simulink model "LinearVehicleiLQR"  (R2021a)
settings: Solver=FixedStepDiscrete  StartTime=0.0  StopTime=100  FixedStep=0.001  MaxStep=0.01  RelTol=1e-3
values from neighbouring files (symbols this model uses):
  Q = [1 0 0; 0 1 0; 0 0 10]    [LQR.m]    (also in NonlinearVehicleLQR.m = eye(3)*10; NonlinearVehicleiLQR.m = eye(3)*10; SringiLQR.m = [1 0; 0 1]*1; SringiLQR2.m = [1 0; 0 1]*1)
  Qf = eye(3)    [LQR.m]    (also in NonlinearVehicleLQR.m; NonlinearVehicleiLQR.m; SringiLQR.m = [1 0; 0 1]; SringiLQR2.m = [1 0; 0 1])
  R = eye(2)*10^-4    [LQR.m]    (also in NonlinearVehicleLQR.m = eye(2)*10^-2; NonlinearVehicleiLQR.m = eye(2)*10^-2; SringiLQR.m = eye(1)*1e-2; SringiLQR2.m = eye(1)*1e-2)
settings Model: Creator=iris  LastModifiedBy=iris
settings SolverCC: AlgebraicLoopSolver=TrustRegion
settings DebuggingCC: SFMachineParentedDataDiag=warning

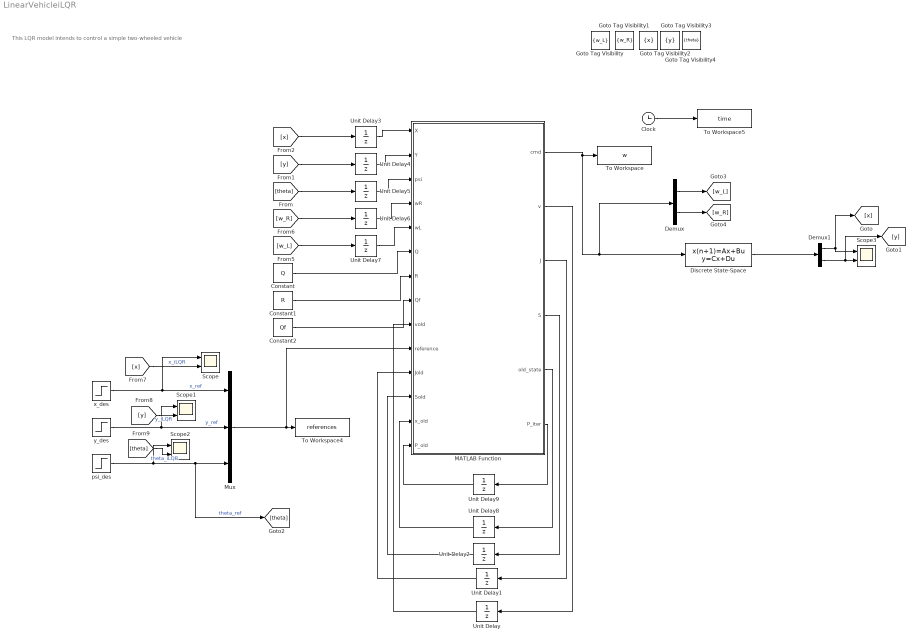
== system LinearVehicleiLQR ==
  note: This LQR model intends to control a simple two-wheeled vehicle
  Clock : Clock
  Constant : Constant  Value=Q
  Constant1 : Constant  Value=R
  Constant2 : Constant  Value=Qf
  Demux : Demux  Outputs=2
  Demux1 : Demux  Outputs=2
  Discrete State-Space : DiscreteStateSpace  A=eye(3)  B=[0.001 0;0 0; 0 0.001]  C=eye(3)  D=zeros(3,2)  SampleTime=-1
  Goto Tag Visibility : GotoTagVisibility  GotoTag=w_L
  Goto Tag Visibility1 : GotoTagVisibility  GotoTag=w_R
  Goto Tag Visibility2 : GotoTagVisibility  GotoTag=x
  Goto Tag Visibility3 : GotoTagVisibility  GotoTag=y
  Goto Tag Visibility4 : GotoTagVisibility  GotoTag=theta
  MATLAB Function : MATLAB Function  TreatAsAtomicUnit=on
  Mux : Mux  Inputs=3
  Scope{,1..3} (4 alike) : Scope  NumInputPorts=2
  To Workspace : ToWorkspace  VariableName=w  SampleTime=-1
  To Workspace4 : ToWorkspace  VariableName=references  SampleTime=-1
  To Workspace5 : ToWorkspace  VariableName=time  SampleTime=-1
  Unit Delay : UnitDelay  InitialCondition=zeros(2,1)  SampleTime=-1  HasFrameUpgradeWarning=on
  Unit Delay1 : UnitDelay  InitialCondition=10000  SampleTime=-1  HasFrameUpgradeWarning=on
  Unit Delay2 : UnitDelay  InitialCondition=Qf  SampleTime=-1  HasFrameUpgradeWarning=on
  Unit Delay{3..7} (5 alike) : UnitDelay  SampleTime=-1  HasFrameUpgradeWarning=on
  Unit Delay8 : UnitDelay  InitialCondition=[0,0]  SampleTime=-1  HasFrameUpgradeWarning=on
  Unit Delay9 : UnitDelay  InitialCondition=zeros(2)  SampleTime=-1  HasFrameUpgradeWarning=on
  psi_des : Step  Time=0  SampleTime=0
  x_des : Step  Time=0  SampleTime=0
  y_des : Step  Time=0  SampleTime=0
  wires:
  MATLAB Function/3(J) -> Unit Delay1/1
  Unit Delay1/1 -> MATLAB Function/11(Jold)
  MATLAB Function/4(S) -> Unit Delay2/1
  Unit Delay2/1 -> MATLAB Function/12(Sold)
  MATLAB Function/2(v) -> Unit Delay/1
  Unit Delay/1 -> MATLAB Function/9(vold)
  MATLAB Function/1(cmd) -> To Workspace/1, Demux/1, Discrete State-Space/1
  [theta] -> Unit Delay5/1
  [x] -> Unit Delay3/1
  [y] -> Unit Delay4/1
  [w_L] -> Unit Delay7/1
  [w_R] -> Unit Delay6/1
  Constant/1 -> MATLAB Function/6(Q)
  Constant1/1 -> MATLAB Function/7(R)
  Constant2/1 -> MATLAB Function/8(Qf)
  Mux/1 -> MATLAB Function/10(reference), To Workspace4/1
  y_des/1 -> Scope1/1, Mux/2  "y_ref"
  x_des/1 -> Mux/1, Scope/1  "x_ref"
  psi_des/1 -> Scope2/1, [theta], Mux/3  "theta_ref"
  Unit Delay3/1 -> MATLAB Function/1(X)
  Unit Delay4/1 -> MATLAB Function/2(Y)
  Unit Delay5/1 -> MATLAB Function/3(psi)
  Unit Delay6/1 -> MATLAB Function/4(wR)
  Unit Delay7/1 -> MATLAB Function/5(wL)
  Clock/1 -> To Workspace5/1
  [x] -> Scope/2  "x_iLQR"
  [y] -> Scope1/2  "y_iLQR"
  [theta] -> Scope2/2  "theta_iLQR"
  Discrete State-Space/1 -> Demux1/1
  Demux1/1 -> [x], Scope3/1
  Demux1/2 -> [y], Scope3/2
  MATLAB Function/5(old_state) -> Unit Delay8/1
  Unit Delay8/1 -> MATLAB Function/13(x_old)
  Demux/1 -> [w_L]
  Demux/2 -> [w_R]
  MATLAB Function/6(P_iter) -> Unit Delay9/1
  Unit Delay9/1 -> MATLAB Function/14(P_old)

== matlab function LinearVehicleiLQR/MATLAB Function ==
  data: X input; cmd output; Y input; psi input; wR input; wL input; Q input; R input; Qf input; vold input; reference input; Jold input; Sold input; v output; J output; S output; old_state output; x_old input; P_old input; P_iter output
function [cmd, v, J, S, old_state, P_iter]= fcn(X, Y, psi, wR, wL, Q, R, Qf, vold, reference, Jold, Sold, x_old, P_old)

r = 0.02;
B = 0.185;
dt = 0.001;

toll = 3*10^-5;

% A = [1 0 dt*-sin(psi)*r/2*(wR+wL);...
%      0 1 dt*cos(psi)*r/2*(wR+wL);...
%      0 0 1];
% B = dt*[cos(psi)*r/2 cos(psi)*r/2;...
%      sin(psi)*r/2 sin(psi)*r/2;...
%      -r/B r/B];
%%% 2i 3o linear model
% % A = eye(3);
% % B = dt*[1 0;...
% %      0 0;...
% %      0 1];
%%% 2i 2o linear model
A = eye(2);
B = eye(2,2);
% A = [1 0 dt*-sin(psi)*r/2*(wR+wL);...
%      0 1 dt*cos(psi)*r/2*(wR+wL);...
%      0 0 1];
% B = dt*[cos(psi)*r/2 cos(psi)*r/2;...
%      sin(psi)*r/2 sin(psi)*r/2;...
%      -r/B r/B];
state = [X Y];
cmd_old = [wL wR];
J = state*Qf*state'+state*Q*state'+cmd_old*R*cmd_old';


% if abs(Jold-J)/Jold > toll
K  = (B'*Sold*B+R)\B'*Sold*A;
Kv = (B'*Sold*B+R)\B';
Ku = (B'*Sold*B+R)\R;
S  = A'*Sold*(A-B*K)+Q;
deltax = -reference(1:length(state));
v  = (A-B*K)'*vold-K'*R*cmd_old'+Q*deltax;
deltau = -K*(x_old'-state)'-Kv*v-Ku*cmd_old';
old_state = state';
% cmd  = cmd_old' + deltau;

%   Alternative from https://people.eecs.berkeley.edu/~pabbeel/cs287-fa12/slides/LQR.pdf
K_iter = -1*(R+B'*P_old*B)\B'*P_old*A;
P_iter = Q + K_iter'*R*K_iter + (A+B*K_iter)'*P_old*(A+B*K_iter);
% %     f = -1*(R+B'*P_old*B)\B'*(P_iter
cmd = K_iter*(deltax);
% else
%     S  = Sold;
%     v  = vold;
%     cmd  = [wL wR]';
%     old_state = state';
end
